simulink model "mpc1v2_1"  (R2020b)
settings: Solver=VariableStepAuto  StartTime=0.0  StopTime=370  RelTol=1e-3
undefined symbols (not defined in the file): Tout2
libraries: dspsrcs4 x2, mpclib x1, cstblocks x1
settings Model: Creator=yanis  LastModifiedBy=yanis

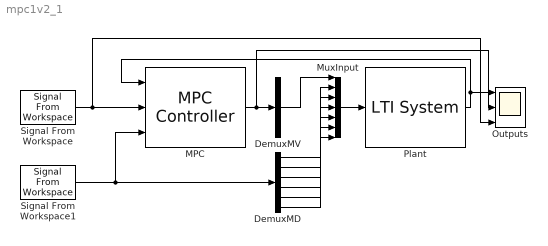
== system mpc1v2_1 ==
  DemuxMD : Demux  Outputs=6
  DemuxMV : Demux  Outputs=1
  MPC : mpclib/MPC Controller  SCDEnableBlockLinearizationSpecification=on  mpcobj=mpc1v2  is_multiple=0  enable_value=0  return_u0=off  updateMPCinCallerWorkspace=on  md_inport=on  mv_inport=off  uref_inport=off  return_cost=off  return_mvseq=off  return_qpstatus=off  return_xseq=off  return_state=off  return_ovseq=off  state_inport=off  umin_inport=off  umax_inport=off  ymin_inport=off  ymax_inport=off  cc_inport=off  ywt_inport=off  uwt_inport=off  duwt_inport=off  rhoeps_inport=off  pm_inport=off  MaximumP=10  HorizonChoice=FixedHorizon  n_ts=0.2  n_p=15  n_mv=1  n_md=6  n_ud=0  n_mo=1  n_uo=0  BlockDataType=double  SampleTimeInherited=off  switch_inport=off
  MuxInput : Mux  Inputs=7
  Outputs : Scope  NumInputPorts=3
  Plant : cstblocks/LTI System  sys=model  IC=[]
  Signal From Workspace : dspsrcs4/Signal From Workspace  X=r  Ts=1  nsamps=1  OutputAfterFinalValue=Setting to zero  ignoreOrWarnInputAndFrameLengths=off  OutputFrames=off
  Signal From Workspace1 : dspsrcs4/Signal From Workspace  X=[Tout2' zeros(length(Tout2), 5)]  Ts=1  nsamps=1  OutputAfterFinalValue=Setting to zero  ignoreOrWarnInputAndFrameLengths=off  OutputFrames=off
  wires:
  Plant/1 -> MPC/1, Outputs/1
  MuxInput/1 -> Plant/1
  MPC/1 -> Outputs/2, DemuxMV/1
  DemuxMV/1 -> MuxInput/1
  Signal From Workspace1/1 -> MPC/3, DemuxMD/1
  DemuxMD/1 -> MuxInput/2
  DemuxMD/2 -> MuxInput/3
  DemuxMD/3 -> MuxInput/4
  DemuxMD/4 -> MuxInput/5
  DemuxMD/5 -> MuxInput/6
  DemuxMD/6 -> MuxInput/7
  Signal From Workspace/1 -> Outputs/3, MPC/2
